simulink model "MAS"  (R2023a)
settings: Solver=FixedStepAuto  StartTime=0.0  StopTime=0.3  FixedStep=1e-6  RelTol=1e-3
values from neighbouring files (symbols this model uses):
  abc_alpha_beta = sqrt(2/3) * [1, -1/2, -1/2 ... (first row only)    [main.m]
  Flux_1 = 1/(Msr^2 - Ls * Lr )  * [Rs*Lr, 0, -Rs*Msr, 0 ... (first row only)    [main.m]
  Flux_2 = 1/(Msr^2 - Ls * Lr )  * [0, 0, 0, 0 ... (first row only)    [main.m]
  frot = 0.01    [main.m]
  Inv_abc_alpha_beta = inv(abc_alpha_beta)    [main.m]
  Inv_Phi_Courant = inv(Phi_Courant)    [main.m]
  J = 0.025    [main.m]
  Lr = 0.194    [main.m]
  Ls = 0.182    [main.m]
  Msr = 0.182    [main.m]
  onduleur = V_MLI/3*[2,-1,-1 ... (first row only)    [main.m]
  p = 2    [main.m]
  Rr = 1.15    [main.m]
  sigma = 1-Msr^2/(Ls*Lr)    (= 0.0618556701031)    [main.m]
  T_charge = 0    [main.m]
  T_MLI = 1/F_MLI    (= 0.0001)    [main.m]
  Trau = T_MLI/(2*pi)    (= 1.59154943092e-05)    [main.m]
  V_MLI = 540    [main.m]
  Vn = 380    [main.m]
  ws = 2*pi*Fn    (= 314.159265359)    [main.m]
libraries: slpidlib x3, simulink x1
settings Model: Creator=philippecasteres  LastModifiedBy=philippecasteres

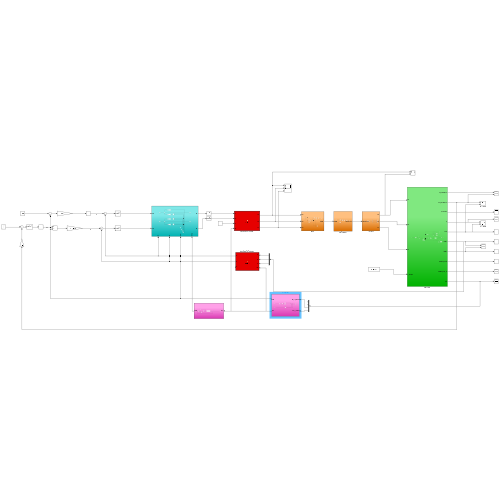
[thumbnail: Simulink's stored preview of the top-level diagram]
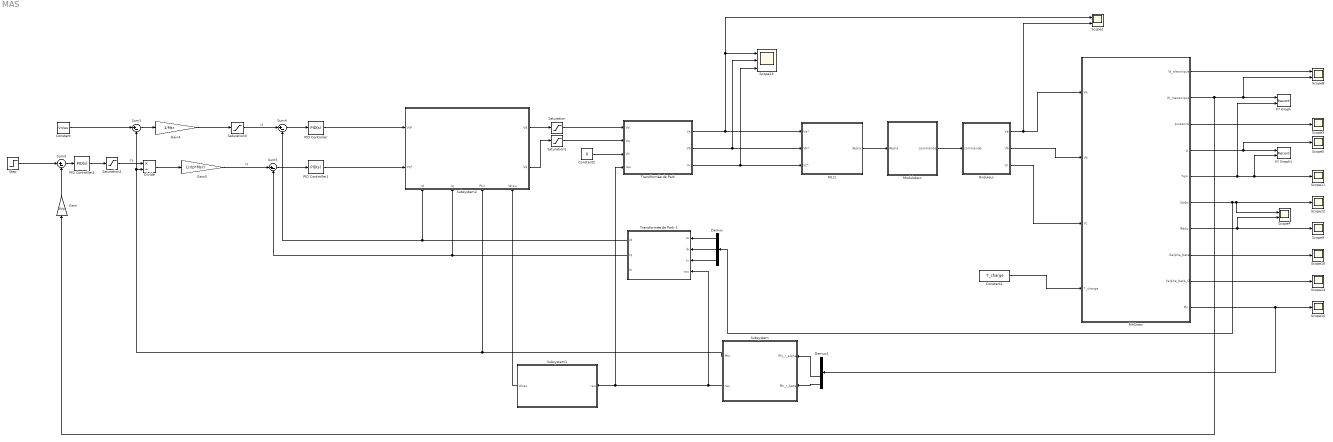
== system MAS ==
  Constant : Constant  Value=Vn/ws
  Constant1 : Constant  Value=T_charge
  Constant2 : Constant  Value=0
  Demux : Demux  Outputs=3
  Demux1 : Demux
  Divide : Product  Inputs=*/
  Gain : Gain  Gain=30/pi
  Gain3 : Gain  Gain=Lr/(p*Msr)
  Gain4 : Gain  Gain=1/Msr
  MASnew : Subsystem
  MLI1 : Subsystem
  Modulateur : Subsystem
  Onduleur : Subsystem
  PID Controller : slpidlib/PID Controller  Controller=PID  Form=Parallel  TimeDomain=Continuous-time  UseExternalTs=off  SampleTime=-1  IntegratorMethod=Forward Euler  FilterMethod=Forward Euler  ControllerParametersSource=internal  P=1  I=1  UseKiTs=off  D=0  N=100  UseFilter=on  TunerSelectOption=Transfer Function Based (PID Tuner App)  InitialConditionSource=internal  InitialConditionForIntegrator=0  InitialConditionForFilter=0  DifferentiatorICPrevScaledInput=0  ExternalReset=none  TrackingMode=off  Kt=1  LimitOutput=off  SatLimitsSource=internal  UpperSaturationLimit=inf  LowerSaturationLimit=-inf  LinearizeAsGain=on  AntiWindupMode=none  Kb=1  LimitIntegrator=off  UpperIntegratorSaturationLimit=inf  LowerIntegratorSaturationLimit=-inf  POutMin=[]  POutMax=[]  IOutMin=[]  IOutMax=[]  DOutMin=[]  DOutMax=[]  NOutMin=[]  NOutMax=[]  SumOutMin=[]  SumOutMax=[]  SaturationOutMin=[]  SaturationOutMax=[]  PParamMin=[]  PParamMax=[]  IParamMin=[]  IParamMax=[]  DParamMin=[]  DParamMax=[]  NParamMin=[]  NParamMax=[]  KbParamMin=[]  KbParamMax=[]  KtParamMin=[]  KtParamMax=[]  KbOutMin=[]  KbOutMax=[]  KtOutMin=[]  KtOutMax=[]  IntegratorOutMin=[]  IntegratorOutMax=[]  FilterOutMin=[]  FilterOutMax=[]  SumI1OutMin=[]  SumI1OutMax=[]  SumI2OutMin=[]  SumI2OutMax=[]  SumI3OutMin=[]  SumI3OutMax=[]  SumI4OutMin=[]  SumI4OutMax=[]  SumDOutMin=[]  SumDOutMax=[]  DifferentiatorOutMin=[]  DifferentiatorOutMax=[]  FilterDiffOutCoefMin=[]  FilterDiffOutCoefMax=[]  ReciprocalOutMin=[]  ReciprocalOutMax=[]  SumDenOutMin=[]  SumDenOutMax=[]  SumNumOutMin=[]  SumNumOutMax=[]  DivideOutMin=[]  DivideOutMax=[]  UdiffTsProdOutMin=[]  UdiffTsProdOutMax=[]  NTsProdOutMin=[]  NTsProdOutMax=[]  UintegralTsProdOutMin=[]  UintegralTsProdOutMax=[]  UngainTsProdOutMin=[]  UngainTsProdOutMax=[]  ClampingZeroOutDataTypeStr=Inherit: Inherit via back propagation  ClampingZeroOutMin=[]  ClampingZeroOutMax=[]  FilterDenConstantOutDataTypeStr=Inherit: Inherit via back propagation  FilterDenConstantOutMin=[]  FilterDenConstantOutMax=[]  PCopyOutDataTypeStr=Inherit: Inherit via back propagation  PCopyOutMin=[]  PCopyOutMax=[]  NCopyOutDataTypeStr=Inherit: Inherit via back propagation  NCopyOutMin=[]  NCopyOutMax=[]  IntegratorContinuousStateAttributes=''  IntegratorStateMustResolveToSignalObject=off  IntegratorRTWStateStorageClass=Auto  FilterContinuousStateAttributes=''  FilterStateMustResolveToSignalObject=off  FilterRTWStateStorageClass=Auto  ParallelPVariant=InternalParameters  IdealPVariant=Disabled  IVariant=InternalParameters  DVariant=InternalParameters  IntegratorVariant=Continuous  SatVariant=Disabled  AWVariant=Passthrough  PCopyVariant=Disabled  TRVariant=Disabled  FdbkBlocksVariant=Forward  IdealPFdbkVariant=Disabled  SatFdbkVariant=Disabled  DerivativeFilterVariant=ContFilter  NVariant=InternalParameters  NCopyVariant=Disabled  FilterICVariant=InternalICsFilter  IntegratorICVariant=InternalICs  ExternalResetVariant=Disabled  TRSumVariant=Passthrough  SumFdbkVariant=Disabled  SumVariant=Sum_PID  TsampFilterVariant=InternalTs  TsampNgainVariant=Passthrough  TsampIntegralVariant=Disabled_SignalSpec  ExternalSaturationOutDataTypeStr=Inherit: Same as second input
  PID Controller1 : slpidlib/PID Controller  Controller=PID  Form=Parallel  TimeDomain=Continuous-time  UseExternalTs=off  SampleTime=-1  IntegratorMethod=Forward Euler  FilterMethod=Forward Euler  ControllerParametersSource=internal  P=1  I=1  UseKiTs=off  D=0  N=100  UseFilter=on  TunerSelectOption=Transfer Function Based (PID Tuner App)  InitialConditionSource=internal  InitialConditionForIntegrator=0  InitialConditionForFilter=0  DifferentiatorICPrevScaledInput=0  ExternalReset=none  TrackingMode=off  Kt=1  LimitOutput=off  SatLimitsSource=internal  UpperSaturationLimit=inf  LowerSaturationLimit=-inf  LinearizeAsGain=on  AntiWindupMode=none  Kb=1  LimitIntegrator=off  UpperIntegratorSaturationLimit=inf  LowerIntegratorSaturationLimit=-inf  POutMin=[]  POutMax=[]  IOutMin=[]  IOutMax=[]  DOutMin=[]  DOutMax=[]  NOutMin=[]  NOutMax=[]  SumOutMin=[]  SumOutMax=[]  SaturationOutMin=[]  SaturationOutMax=[]  PParamMin=[]  PParamMax=[]  IParamMin=[]  IParamMax=[]  DParamMin=[]  DParamMax=[]  NParamMin=[]  NParamMax=[]  KbParamMin=[]  KbParamMax=[]  KtParamMin=[]  KtParamMax=[]  KbOutMin=[]  KbOutMax=[]  KtOutMin=[]  KtOutMax=[]  IntegratorOutMin=[]  IntegratorOutMax=[]  FilterOutMin=[]  FilterOutMax=[]  SumI1OutMin=[]  SumI1OutMax=[]  SumI2OutMin=[]  SumI2OutMax=[]  SumI3OutMin=[]  SumI3OutMax=[]  SumI4OutMin=[]  SumI4OutMax=[]  SumDOutMin=[]  SumDOutMax=[]  DifferentiatorOutMin=[]  DifferentiatorOutMax=[]  FilterDiffOutCoefMin=[]  FilterDiffOutCoefMax=[]  ReciprocalOutMin=[]  ReciprocalOutMax=[]  SumDenOutMin=[]  SumDenOutMax=[]  SumNumOutMin=[]  SumNumOutMax=[]  DivideOutMin=[]  DivideOutMax=[]  UdiffTsProdOutMin=[]  UdiffTsProdOutMax=[]  NTsProdOutMin=[]  NTsProdOutMax=[]  UintegralTsProdOutMin=[]  UintegralTsProdOutMax=[]  UngainTsProdOutMin=[]  UngainTsProdOutMax=[]  ClampingZeroOutDataTypeStr=Inherit: Inherit via back propagation  ClampingZeroOutMin=[]  ClampingZeroOutMax=[]  FilterDenConstantOutDataTypeStr=Inherit: Inherit via back propagation  FilterDenConstantOutMin=[]  FilterDenConstantOutMax=[]  PCopyOutDataTypeStr=Inherit: Inherit via back propagation  PCopyOutMin=[]  PCopyOutMax=[]  NCopyOutDataTypeStr=Inherit: Inherit via back propagation  NCopyOutMin=[]  NCopyOutMax=[]  IntegratorContinuousStateAttributes=''  IntegratorStateMustResolveToSignalObject=off  IntegratorRTWStateStorageClass=Auto  FilterContinuousStateAttributes=''  FilterStateMustResolveToSignalObject=off  FilterRTWStateStorageClass=Auto  ParallelPVariant=InternalParameters  IdealPVariant=Disabled  IVariant=InternalParameters  DVariant=InternalParameters  IntegratorVariant=Continuous  SatVariant=Disabled  AWVariant=Passthrough  PCopyVariant=Disabled  TRVariant=Disabled  FdbkBlocksVariant=Forward  IdealPFdbkVariant=Disabled  SatFdbkVariant=Disabled  DerivativeFilterVariant=ContFilter  NVariant=InternalParameters  NCopyVariant=Disabled  FilterICVariant=InternalICsFilter  IntegratorICVariant=InternalICs  ExternalResetVariant=Disabled  TRSumVariant=Passthrough  SumFdbkVariant=Disabled  SumVariant=Sum_PID  TsampFilterVariant=InternalTs  TsampNgainVariant=Passthrough  TsampIntegralVariant=Disabled_SignalSpec  ExternalSaturationOutDataTypeStr=Inherit: Same as second input
  PID Controller2 : slpidlib/PID Controller  Controller=PID  Form=Parallel  TimeDomain=Continuous-time  UseExternalTs=off  SampleTime=-1  IntegratorMethod=Forward Euler  FilterMethod=Forward Euler  ControllerParametersSource=internal  P=1  I=1  UseKiTs=off  D=0  N=100  UseFilter=on  TunerSelectOption=Transfer Function Based (PID Tuner App)  InitialConditionSource=internal  InitialConditionForIntegrator=0  InitialConditionForFilter=0  DifferentiatorICPrevScaledInput=0  ExternalReset=none  TrackingMode=off  Kt=1  LimitOutput=off  SatLimitsSource=internal  UpperSaturationLimit=inf  LowerSaturationLimit=-inf  LinearizeAsGain=on  AntiWindupMode=none  Kb=1  LimitIntegrator=off  UpperIntegratorSaturationLimit=inf  LowerIntegratorSaturationLimit=-inf  POutMin=[]  POutMax=[]  IOutMin=[]  IOutMax=[]  DOutMin=[]  DOutMax=[]  NOutMin=[]  NOutMax=[]  SumOutMin=[]  SumOutMax=[]  SaturationOutMin=[]  SaturationOutMax=[]  PParamMin=[]  PParamMax=[]  IParamMin=[]  IParamMax=[]  DParamMin=[]  DParamMax=[]  NParamMin=[]  NParamMax=[]  KbParamMin=[]  KbParamMax=[]  KtParamMin=[]  KtParamMax=[]  KbOutMin=[]  KbOutMax=[]  KtOutMin=[]  KtOutMax=[]  IntegratorOutMin=[]  IntegratorOutMax=[]  FilterOutMin=[]  FilterOutMax=[]  SumI1OutMin=[]  SumI1OutMax=[]  SumI2OutMin=[]  SumI2OutMax=[]  SumI3OutMin=[]  SumI3OutMax=[]  SumI4OutMin=[]  SumI4OutMax=[]  SumDOutMin=[]  SumDOutMax=[]  DifferentiatorOutMin=[]  DifferentiatorOutMax=[]  FilterDiffOutCoefMin=[]  FilterDiffOutCoefMax=[]  ReciprocalOutMin=[]  ReciprocalOutMax=[]  SumDenOutMin=[]  SumDenOutMax=[]  SumNumOutMin=[]  SumNumOutMax=[]  DivideOutMin=[]  DivideOutMax=[]  UdiffTsProdOutMin=[]  UdiffTsProdOutMax=[]  NTsProdOutMin=[]  NTsProdOutMax=[]  UintegralTsProdOutMin=[]  UintegralTsProdOutMax=[]  UngainTsProdOutMin=[]  UngainTsProdOutMax=[]  ClampingZeroOutDataTypeStr=Inherit: Inherit via back propagation  ClampingZeroOutMin=[]  ClampingZeroOutMax=[]  FilterDenConstantOutDataTypeStr=Inherit: Inherit via back propagation  FilterDenConstantOutMin=[]  FilterDenConstantOutMax=[]  PCopyOutDataTypeStr=Inherit: Inherit via back propagation  PCopyOutMin=[]  PCopyOutMax=[]  NCopyOutDataTypeStr=Inherit: Inherit via back propagation  NCopyOutMin=[]  NCopyOutMax=[]  IntegratorContinuousStateAttributes=''  IntegratorStateMustResolveToSignalObject=off  IntegratorRTWStateStorageClass=Auto  FilterContinuousStateAttributes=''  FilterStateMustResolveToSignalObject=off  FilterRTWStateStorageClass=Auto  ParallelPVariant=InternalParameters  IdealPVariant=Disabled  IVariant=InternalParameters  DVariant=InternalParameters  IntegratorVariant=Continuous  SatVariant=Disabled  AWVariant=Passthrough  PCopyVariant=Disabled  TRVariant=Disabled  FdbkBlocksVariant=Forward  IdealPFdbkVariant=Disabled  SatFdbkVariant=Disabled  DerivativeFilterVariant=ContFilter  NVariant=InternalParameters  NCopyVariant=Disabled  FilterICVariant=InternalICsFilter  IntegratorICVariant=InternalICs  ExternalResetVariant=Disabled  TRSumVariant=Passthrough  SumFdbkVariant=Disabled  SumVariant=Sum_PID  TsampFilterVariant=InternalTs  TsampNgainVariant=Passthrough  TsampIntegralVariant=Disabled_SignalSpec  ExternalSaturationOutDataTypeStr=Inherit: Same as second input
  Saturation{,1..3} (4 alike) : Saturate
  Scope{3,5,9..12,14..15} (8 alike) : Scope
  Scope13 : Scope  NumInputPorts=3
  Scope2 : Scope  NumInputPorts=2
  Scope4 : Scope  NumInputPorts=2
  Scope8 : Scope  NumInputPorts=2
  Step : Step  Time=0.1  SampleTime=0
  Subsystem : Subsystem
  Subsystem1 : Subsystem
  Subsystem2 : Subsystem
      settings: PortSchema="{\"entries\":[{\"content\":{\"sides\":[{\"content\":{\"connectorIds\":[\"In1\",\"In2\"]},\"type\":\"ConnectorPlacement.EquallySpacedRectSide\",\"uuid\":\"374a3029-9c19-44eb-9b98-de55e62c7022\"},{\"content\":{\"connectorIds\":[\"Out1\",\"Out2\"],\"side\":\"RIGHT\"},\"type\":\"ConnectorPlacement.EquallySpacedRectSide\",\"uuid\":\"b066ba17-ce68-41f6-a300-7d3bc4dc3f92\"},{\"content\":{\"side\":\"TOP\"},\"type\":\"ConnectorPlacement.EquallySpacedRectSide\",\"uuid\":\"ed738241-ae45-464d-a05c-a5861c3f77ca\"},{\"content\":{\"connectorIds\":[\"In3\",\"In4\",\"In5\",\"In6\"],\"side\":\"BOTTOM\"},\"type\":\"ConnectorPlacement.EquallySpacedRectSide\",\"uuid\":\"e5249242-5c32-4682-b932-0c2aba441929\"}]},\"type\":\"ConnectorPlacement.EquallySpacedConnector\",\"uuid\":\"519ae50f-d565-4f6e-aabe-7acf3d791e4a\"}],\"packageUris\":[\"http://schema.mathworks.com/mf0/Connector/R2020b\"],\"version\":\"1.0\"}"
  Sum{1,3..5} (4 alike) : Sum  Inputs=|+-
  Transformée de Park : MATLAB Function  TreatAsAtomicUnit=on
  Transformée de Park-1 : MATLAB Function  TreatAsAtomicUnit=on
  XY Graph : Record  FileSettingsInternal="{\"entries\":[{\"content\":{\"excelSettings\":{\"content\":{},\"type\":\"Streamout.ExcelSettings\"}},\"type\":\"Streamout.FileSettingStorage\",\"uuid\":\"f28bcfdc-29c8-41b2-9037-532fc5c7e8b2\"}],\"packageUris\":[\"http://schema.mathworks.com/mf0/streamout_blocks/R2020a\"],\"version\":\"1.0\"}"  Layout=[1 1]  SignalsInternal="{\"entries\":[{\"content\":{\"signals\":[{\"content\":{\"blockPath\":[\"MAS/XY Graph\"],\"dimensions\":[1],\"domain\":\"MAS/XY Graph\",\"lineColor\":\"#a2142f\",\"plots\":[1],\"port\":1,\"sid\":[\"\"],\"signalID\":4156,\"signalName\":\"MASnew:2\"},\"type\":\"RecordBlkView.Signal\",\"uuid\":\"834b7e5b-c07c-4418-9d5a-896b98f5fa33\"},{\"content\":{\"blockPath\":[\"MAS/XY Graph\"],\"dimensions\":[1],\"domain\":\"MAS/XY Graph\",\"lineColor\":\"#139fff\",\"plots\":[1],\"port\":2,\"sid\":[\"\"],\"signalID\":4160,\"signalName\":\"MASnew:5\"},\"type\":\"RecordBlkView.Signal\",\"uuid\":\"b30b5f0e-b342-480d-b9e4-c4c33390f40f\"}]},\"type\":\"RecordBlkView.InputSignals\",\"uuid\":\"d0d9e1e5-2b0f-47f1-a562-6059a6d6e037\"}],\"packageUris\":[\"http://schema.mathworks.com/mf0/streamout_blocks/R2020a\"],\"version\":\"1.0\"}"  VisualizationBindings="{\"xyplotplugin\":{\"info\":[{\"series\":[{\"bindingParametersList\":[{\"parameter\":\"X-Axis\",\"signalID\":4156,\"signalName\":\"MASnew:2\"},{\"parameter\":\"Y-Axis\",\"signalID\":4160,\"signalName\":\"MASnew:5\"}],\"seriesID\":49409}],\"subplotID\":1}]}}"  CompatibilityTag=XY
  XY Graph1 : Record  FileSettingsInternal="{\"entries\":[{\"content\":{\"excelSettings\":{\"content\":{},\"type\":\"Streamout.ExcelSettings\"}},\"type\":\"Streamout.FileSettingStorage\",\"uuid\":\"aadc846a-b6cb-4434-9563-fc8bc5a6f5f1\"}],\"packageUris\":[\"http://schema.mathworks.com/mf0/streamout_blocks/R2020a\"],\"version\":\"1.0\"}"  Layout=[1 1]  SignalsInternal="{\"entries\":[{\"content\":{\"signals\":[{\"content\":{\"blockPath\":[\"MAS/XY Graph1\"],\"dimensions\":[1],\"domain\":\"MAS/XY Graph1\",\"lineColor\":\"#a2142f\",\"plots\":[1],\"port\":1,\"sid\":[\"\"],\"signalID\":4164,\"signalName\":\"MASnew:4\"},\"type\":\"RecordBlkView.Signal\",\"uuid\":\"23fc42c7-f1db-4600-8dec-494fe7667da3\"},{\"content\":{\"blockPath\":[\"MAS/XY Graph1\"],\"dimensions\":[1],\"domain\":\"MAS/XY Graph1\",\"lineColor\":\"#139fff\",\"plots\":[1],\"port\":2,\"sid\":[\"\"],\"signalID\":4168,\"signalName\":\"MASnew:5\"},\"type\":\"RecordBlkView.Signal\",\"uuid\":\"0e7de400-2c3a-4ac4-9282-795aee7cb059\"}]},\"type\":\"RecordBlkView.InputSignals\",\"uuid\":\"fc30f45e-be68-4fd3-a892-06cb04b79526\"}],\"packageUris\":[\"http://schema.mathworks.com/mf0/streamout_blocks/R2020a\"],\"version\":\"1.0\"}"  VisualizationBindings="{\"xyplotplugin\":{\"info\":[{\"series\":[{\"bindingParametersList\":[{\"parameter\":\"X-Axis\",\"signalID\":4164,\"signalName\":\"MASnew:4\"},{\"parameter\":\"Y-Axis\",\"signalID\":4168,\"signalName\":\"MASnew:5\"}],\"seriesID\":17936}],\"subplotID\":1}]}}"  CompatibilityTag=XY
  wires:
  Demux/1 -> Transformée de Park-1/1(Ia)
  Demux/2 -> Transformée de Park-1/2(Ib)
  Demux/3 -> Transformée de Park-1/3(Ic)
  Constant1/1 -> MASnew/4(T_charge)
  Transformée de Park/2(Vb) -> MLI1/2(Vb*), Scope13/2
  Onduleur/1(Va) -> MASnew/1(Va), Scope2/2
  Transformée de Park/3(Vc) -> MLI1/3(Vc*), Scope13/3
  MASnew/8(ISalpha_beta) -> Scope10/1
  MASnew/3(puisance) -> Scope3/1
  MASnew/6(ISabc) -> Demux/1, Scope12/1, Scope4/1
  MASnew/7(IRabc) -> Scope4/2, Scope9/1
  Transformée de Park/1(Va) -> MLI1/1(Va*), Scope13/1, Scope2/1
  MASnew/2(W_mecanique) -> Gain/1, Scope8/2, XY Graph/1
  MASnew/1(W_electrique) -> Scope8/1
  MASnew/5(Tem) -> XY Graph/2, XY Graph1/2, Scope11/1
  MASnew/4(g) -> Scope5/1, XY Graph1/1
  MASnew/9(Valpha_beta_O) -> Scope14/1
  MASnew/10(Phi) -> Demux1/1, Scope15/1
  Onduleur/3(Vc) -> MASnew/3(Vc)
  Onduleur/2(Vb) -> MASnew/2(Vb)
  Sum4/1 -> PID Controller/1
  Transformée de Park-1/1(Id) -> Sum4/2, Subsystem2/3(Id)
  Sum5/1 -> PID Controller1/1
  Saturation3/1 -> Sum4/1  "Id"
  Gain3/1 -> Sum5/1  "Iq"
  Transformée de Park-1/2(Iq) -> Sum5/2, Subsystem2/4(Iq)
  Demux1/3 -> Subsystem/1(Phi_r_alpha)
  Demux1/4 -> Subsystem/2(Phi_r_beta)
  Subsystem/2(rau) -> Transformée de Park/4(rau), Subsystem1/1(rau), Transformée de Park-1/4(rau)
  Saturation/1 -> Transformée de Park/1(Vd)
  Saturation1/1 -> Transformée de Park/2(Vq)
  Divide/1 -> Gain3/1
  Saturation2/1 -> Divide/1  "Ce"
  Gain4/1 -> Saturation3/1
  Subsystem/1(Phir) -> Divide/2, Sum1/2, Subsystem2/5(Phir)
  Sum1/1 -> Gain4/1
  PID Controller2/1 -> Saturation2/1
  Sum3/1 -> PID Controller2/1
  Modulateur/1(commande) -> Onduleur/1(commande)
  MLI1/1(Alpha) -> Modulateur/1(Alpha)
  PID Controller/1 -> Subsystem2/1(Vd*)
  PID Controller1/1 -> Subsystem2/2(Vq*)
  Subsystem1/1(Wrau) -> Subsystem2/6(Wrau)
  Subsystem2/1(Vd) -> Saturation/1
  Subsystem2/2(Vq) -> Saturation1/1
  Gain/1 -> Sum3/2
  Step/1 -> Sum3/1
  Constant/1 -> Sum1/1
  Constant2/1 -> Transformée de Park/3(Vh)

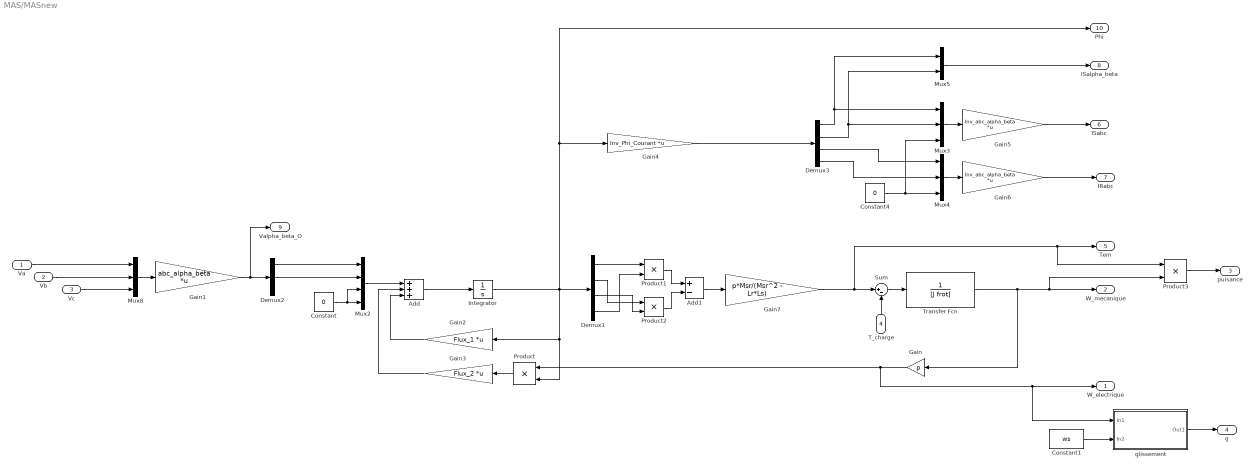
== system MAS/MASnew ==
  Va : Inport
  Vb : Inport  Port=2
  Vc : Inport  Port=3
  T_charge : Inport  Port=4
  Add : Sum  Inputs=+++
  Add1 : Sum  Inputs=+-
  Constant : Constant  Value=0
  Constant1 : Constant  Value=ws
  Constant4 : Constant  Value=0
  Demux1 : Demux
  Demux2 : Demux  Outputs=3
  Demux3 : Demux
  Gain : Gain  Gain=p
  Gain1 : Gain  Gain=abc_alpha_beta  Multiplication=Matrix(K*u)
  Gain2 : Gain  Gain=Flux_1  Multiplication=Matrix(K*u)
  Gain3 : Gain  Gain=Flux_2  Multiplication=Matrix(K*u)
  Gain4 : Gain  Gain=Inv_Phi_Courant  Multiplication=Matrix(K*u)
  Gain5 : Gain  Gain=Inv_abc_alpha_beta  Multiplication=Matrix(K*u)
  Gain6 : Gain  Gain=Inv_abc_alpha_beta  Multiplication=Matrix(K*u)
  Gain7 : Gain  Gain=p*Msr/(Msr^2 - Lr*Ls)
  Integrator : Integrator
  Mux2 : Mux
  Mux3 : Mux  Inputs=3
  Mux4 : Mux  Inputs=3
  Mux5 : Mux  Inputs=2
  Mux8 : Mux  Inputs=3
  Product{,1..3} (4 alike) : Product
  Sum : Sum  Inputs=|+-
  Transfer Fcn : TransferFcn  Denominator=[J frot]
  glissement : Subsystem
  W_electrique : Outport
  W_mecanique : Outport  Port=2
  puisance : Outport  Port=3
  g : Outport  Port=4
  Tem : Outport  Port=5
  ISabc : Outport  Port=6
  IRabc : Outport  Port=7
  ISalpha_beta : Outport  Port=8
  Valpha_beta_O : Outport  Port=9
  Phi : Outport  Port=10
  wires:
  Demux3/4 -> Mux4/2
  Demux3/2 -> Mux3/2, Mux5/2
  T_charge/1 -> Sum/2
  Demux3/1 -> Mux3/1, Mux5/1
  Va/1 -> Mux8/1
  Sum/1 -> Transfer Fcn/1
  Demux1/1 -> Product1/1
  Demux3/3 -> Mux4/1
  Gain7/1 -> Sum/1, Product3/1, Tem/1
  Transfer Fcn/1 -> Gain/1, Product3/2, W_mecanique/1
  Add/1 -> Integrator/1
  Vc/1 -> Mux8/3
  Vb/1 -> Mux8/2
  Product/1 -> Gain3/1
  Integrator/1 -> Gain2/1, Product/2, Demux1/1, Gain4/1, Phi/1
  Mux2/1 -> Add/1
  Mux3/1 -> Gain5/1
  Mux5/1 -> ISalpha_beta/1
  Gain1/1 -> Valpha_beta_O/1, Demux2/1
  Mux8/1 -> Gain1/1
  Demux2/1 -> Mux2/1
  Demux2/2 -> Mux2/2
  Constant/1 -> Mux2/4, Mux2/3
  Gain2/1 -> Add/3
  Gain4/1 -> Demux3/1
  Constant4/1 -> Mux4/3, Mux3/3
  Gain5/1 -> ISabc/1
  Mux4/1 -> Gain6/1
  Gain6/1 -> IRabc/1
  Product1/1 -> Add1/1
  Product2/1 -> Add1/2
  Add1/1 -> Gain7/1
  Gain/1 -> glissement/1(In1), W_electrique/1, Product/1
  Gain3/1 -> Add/2
  Demux1/4 -> Product1/2
  Demux1/2 -> Product2/1
  Demux1/3 -> Product2/2
  Product3/1 -> puisance/1
  glissement/1(Out1) -> g/1
  Constant1/1 -> glissement/2(In2)

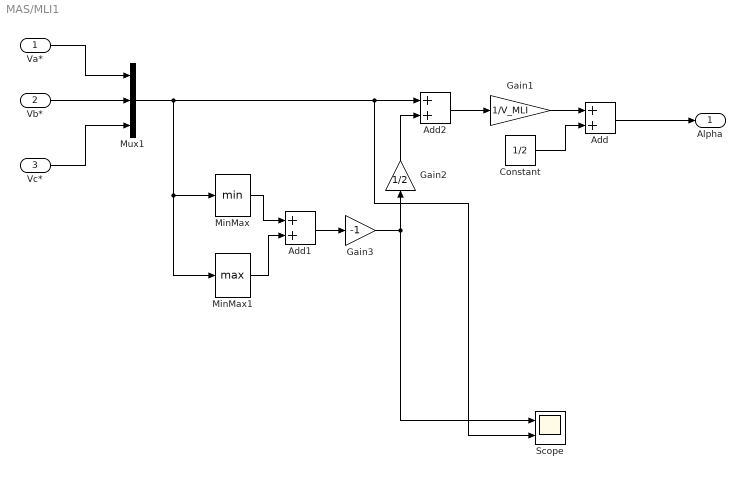
== system MAS/MLI1 ==
  Va* : Inport
  Vb* : Inport  Port=2
  Vc* : Inport  Port=3
  Add : Sum
  Add1 : Sum
  Add2 : Sum
  Constant : Constant  Value=1/2
  Gain1 : Gain  Gain=1/V_MLI
  Gain2 : Gain  Gain=1/2
  Gain3 : Gain  Gain=-1
  MinMax : MinMax
  MinMax1 : MinMax  Function=max
  Mux1 : Mux  Inputs=3
  Scope : Scope  NumInputPorts=2
  Alpha : Outport
  wires:
  Va*/1 -> Mux1/1
  Gain1/1 -> Add/1
  Vb*/1 -> Mux1/2
  Vc*/1 -> Mux1/3
  Add/1 -> Alpha/1
  Add2/1 -> Gain1/1
  Constant/1 -> Add/2
  Gain2/1 -> Add2/2
  Mux1/1 -> Add2/1, Scope/2, MinMax/1, MinMax1/1
  Add1/1 -> Gain3/1
  MinMax/1 -> Add1/1
  MinMax1/1 -> Add1/2
  Gain3/1 -> Scope/1, Gain2/1

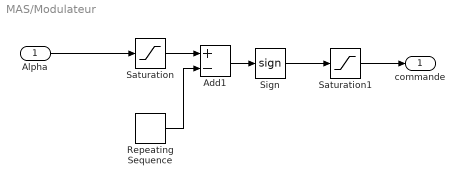
== system MAS/Modulateur ==
  Alpha : Inport
  Add1 : Sum  Inputs=+-
  Repeating Sequence : simulink/Sources/Repeating Sequence  rep_seq_t=[0 0.5*T_MLI T_MLI]  rep_seq_y=[1 0 1]
  Saturation : Saturate  UpperLimit=1  LowerLimit=0
  Saturation1 : Saturate  UpperLimit=1  LowerLimit=0
  Sign : Signum
  commande : Outport
  wires:
  Alpha/1 -> Saturation/1
  Repeating Sequence/1 -> Add1/2
  Add1/1 -> Sign/1
  Sign/1 -> Saturation1/1
  Saturation/1 -> Add1/1
  Saturation1/1 -> commande/1

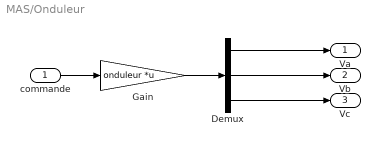
== system MAS/Onduleur ==
  commande : Inport
  Demux : Demux  Outputs=3
  Gain : Gain  Gain=onduleur  Multiplication=Matrix(K*u)
  Va : Outport
  Vb : Outport  Port=2
  Vc : Outport  Port=3
  wires:
  Gain/1 -> Demux/1
  commande/1 -> Gain/1
  Demux/3 -> Vc/1
  Demux/1 -> Va/1
  Demux/2 -> Vb/1

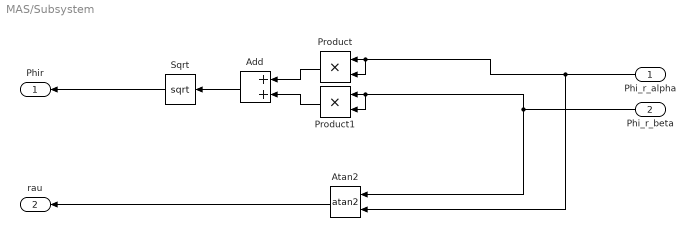
== system MAS/Subsystem ==
  Phi_r_alpha : Inport
  Phi_r_beta : Inport  Port=2
  Add : Sum
  Atan2 : Trigonometry  Operator=atan2
  Product : Product
  Product1 : Product
  Sqrt : Sqrt
  Phir : Outport
  rau : Outport  Port=2
  wires:
  Atan2/1 -> rau/1
  Sqrt/1 -> Phir/1
  Product1/1 -> Add/2
  Add/1 -> Sqrt/1
  Phi_r_beta/1 -> Atan2/1, Product1/2, Product1/1
  Product/1 -> Add/1
  Phi_r_alpha/1 -> Atan2/2, Product/2, Product/1

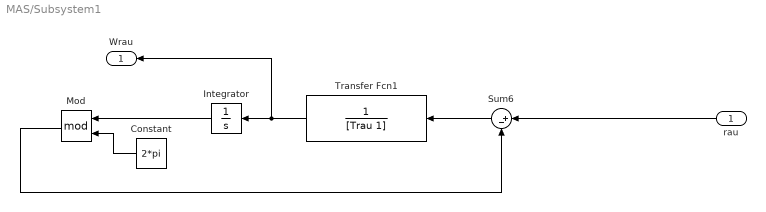
== system MAS/Subsystem1 ==
  rau : Inport
  Constant : Constant  Value=2*pi
  Integrator : Integrator
  Mod : Math  Operator=mod
  Sum6 : Sum  Inputs=|+-
  Transfer Fcn1 : TransferFcn  Denominator=[Trau 1]
  Wrau : Outport
  wires:
  Constant/1 -> Mod/2
  Integrator/1 -> Mod/1
  Mod/1 -> Sum6/2
  Transfer Fcn1/1 -> Wrau/1, Integrator/1
  rau/1 -> Sum6/1
  Sum6/1 -> Transfer Fcn1/1

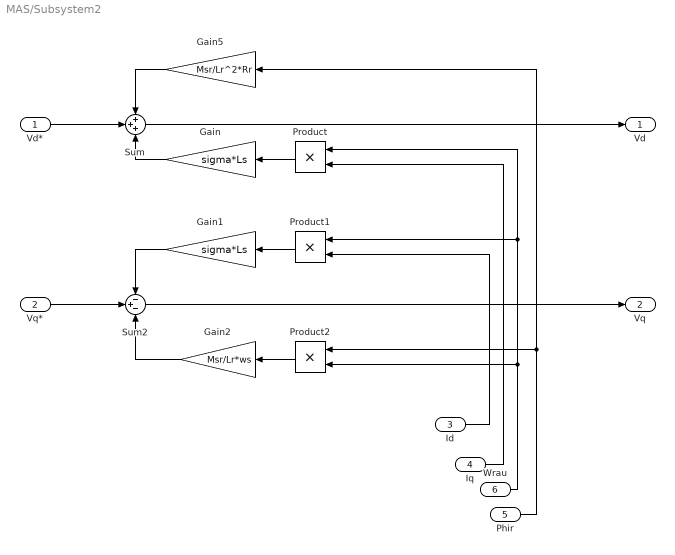
== system MAS/Subsystem2 ==
  Vd* : Inport
  Vq* : Inport  Port=2
  Id : Inport  Port=3
  Iq : Inport  Port=4
  Phir : Inport  Port=5
  Wrau : Inport  Port=6
  Gain : Gain  Gain=sigma*Ls
  Gain1 : Gain  Gain=sigma*Ls
  Gain2 : Gain  Gain=Msr/Lr*ws
  Gain5 : Gain  Gain=Msr/Lr^2*Rr
  Product : Product
  Product1 : Product
  Product2 : Product
  Sum : Sum  Inputs=+++
  Sum2 : Sum  Inputs=-+-
  Vd : Outport
  Vq : Outport  Port=2
  wires:
  Vd*/1 -> Sum/2
  Iq/1 -> Product/2
  Id/1 -> Product1/2
  Gain/1 -> Sum/3
  Product/1 -> Gain/1
  Gain1/1 -> Sum2/1
  Product1/1 -> Gain1/1
  Vq*/1 -> Sum2/2
  Wrau/1 -> Product2/2, Product1/1, Product/1
  Phir/1 -> Product2/1, Gain5/1
  Gain5/1 -> Sum/1
  Sum2/1 -> Vq/1
  Product2/1 -> Gain2/1
  Sum/1 -> Vd/1
  Gain2/1 -> Sum2/3

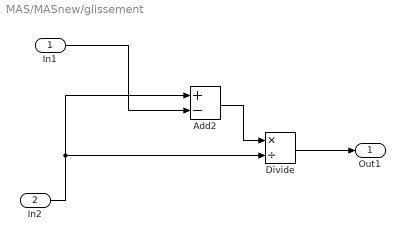
== system MAS/MASnew/glissement ==
  In1 : Inport
  In2 : Inport  Port=2
  Add2 : Sum  Inputs=+-
  Divide : Product  Inputs=*/
  Out1 : Outport
  wires:
  In2/1 -> Divide/2, Add2/1
  Divide/1 -> Out1/1
  In1/1 -> Add2/2
  Add2/1 -> Divide/1

== matlab function MAS/Transformée de Park ==
  data: Vd input; Va output; Vb output; Vc output; Vq input; Vh input; rau input
function [Va, Vb, Vc] = dq_abc(Vd,Vq,Vh,rau)


    % Vecteur de tensions d'entrée
    V = [Vd;Vq;Vh];
    
    % Matrice de transformation
    transformation_matrix = sqrt(2/3) * [cos(rau), cos(rau - 2*pi/3), cos(rau + 2*pi/3);
                                         -sin(rau), -sin(rau - 2*pi/3), -sin(rau + 2*pi/3);
                                          1/sqrt(2), 1/sqrt(2), 1/sqrt(2)];
    
    % Calcul des résultats
    result = transformation_matrix * V;
    
    % Attribution des résultats aux sorties
    Va = result(1);
    Vb= result(2);
    Vc = result(3);




end

== matlab function MAS/Transformée de Park-1 ==
  data: Ia input; Id output; Iq output; Ih output; Ib input; Ic input; rau input
function [Id,Iq,Ih] = dq_abc(Ia, Ib, Ic,rau)


    % Vecteur de tensions d'entrée
    I = [Ia; Ib; Ic];
    
    % Matrice de transformation
    transformation_matrix = sqrt(2/3) * [cos(rau), cos(rau - 2*pi/3), cos(rau + 2*pi/3);
                                         -sin(rau), -sin(rau - 2*pi/3), -sin(rau + 2*pi/3);
                                          1/sqrt(2), 1/sqrt(2), 1/sqrt(2)];
    
    % Calcul des résultats
    result = inv(transformation_matrix) * I;
    
    % Attribution des résultats aux sorties
    Id = result(1);
    Iq= result(2);
    Ih = result(3);




end
